simulink model "variacion_n"  (R2019b)
settings: Solver=VariableStepAuto  StartTime=0.0  StopTime=15000  RelTol=1e-3
undefined symbols (not defined in the file): n, nAum, nDis, nMitadDis, p1, p2, p3, Vi
libraries: simulink x4
settings Model: Creator=USUARIO  LastModifiedBy=USUARIO

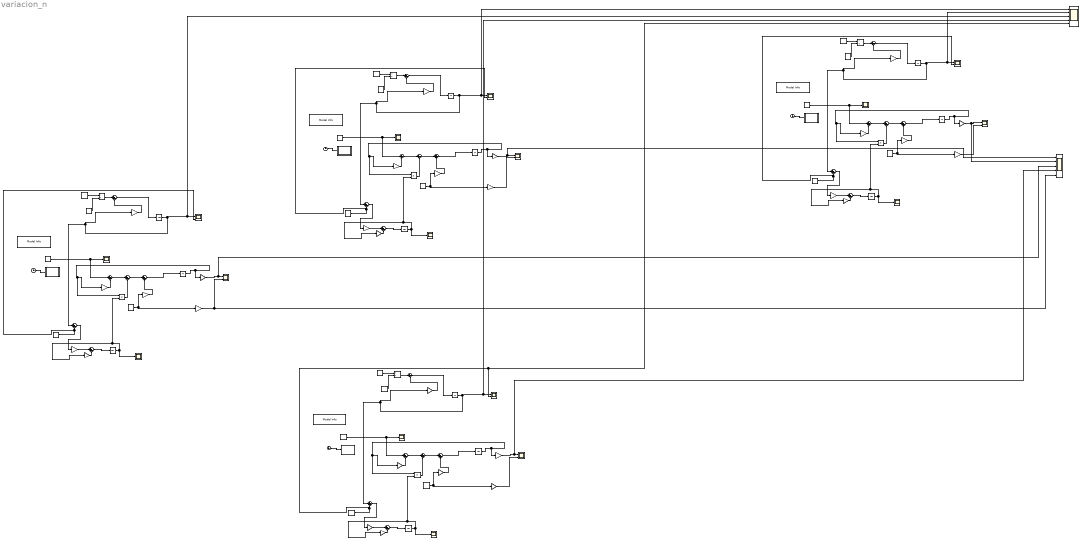
== system variacion_n ==
  Clock{1..4} (4 alike) : Clock
  Constant{1,3,5..6} (4 alike) : Constant  Value=0
  Constant{2,4,7..8} (4 alike) : Constant  Value=Vi
  Divide{1..4} (4 alike) : Product  Inputs=*/
  Gain{1,6,8,13..14,19,22,27} (8 alike) : Gain  Gain=p1
  Gain{3,5,10,12,16,18,24,26} (8 alike) : Gain  Gain=18
  Gain11 : Gain  Gain=nAum
  Gain{2,9,15,23} (4 alike) : Gain  Gain=p3
  Gain17 : Gain  Gain=n
  Gain{7,20..21,28} (4 alike) : Gain  Gain=p2
  Gain25 : Gain  Gain=nMitadDis
  Gain4 : Gain  Gain=nDis
  Glucosa basal{1..4} (4 alike) : Constant  Value=7
  Grafica ingesta D{1..4} (4 alike) : Scope
  Ingesta 75 g1 : MATLAB Function  TreatAsAtomicUnit=on
  Ingesta 75 g2 : MATLAB Function  TreatAsAtomicUnit=on
  Ingesta 75 g3 : MATLAB Function  TreatAsAtomicUnit=on
  Ingesta 75 g4 : MATLAB Function  TreatAsAtomicUnit=on
  Insulina basal{1..4} (4 alike) : Constant  Value=10
  Integrator{1,4,7,10} (4 alike) : Integrator  InitialCondition=10
  Integrator{2,5,8,11} (4 alike) : Integrator  InitialCondition=7
  Integrator{3,6,9,12} (4 alike) : Integrator  InitialCondition=-0.000194
  Model Info1 : simulink/Model-Wide Utilities/Model Info  Frame=on  DisplayStringWithTags=|  HorizontalTextAlignment=Center  LeftAlignmentValue=0.5
      | MODELO MODIFICADO
      | 
      | TRAS INGESTA CON INSULINA
      | 
      | PERSONA DIABETICA
  Model Info2 : simulink/Model-Wide Utilities/Model Info  Frame=on  DisplayStringWithTags=|  HorizontalTextAlignment=Center  LeftAlignmentValue=0.5
      | MODELO MODIFICADO
      | 
      | TRAS INGESTA CON INSULINA
      | 
      | PERSONA DIABETICA
  Model Info3 : simulink/Model-Wide Utilities/Model Info  Frame=on  DisplayStringWithTags=|  HorizontalTextAlignment=Center  LeftAlignmentValue=0.5
      | MODELO MODIFICADO
      | 
      | TRAS INGESTA CON INSULINA
      | 
      | PERSONA DIABETICA
  Model Info4 : simulink/Model-Wide Utilities/Model Info  Frame=on  DisplayStringWithTags=|  HorizontalTextAlignment=Center  LeftAlignmentValue=0.5
      | MODELO MODIFICADO
      | 
      | TRAS INGESTA CON INSULINA
      | 
      | PERSONA DIABETICA
  Product{1..4} (4 alike) : Product
  Sum{1..2,4..8,10..15,17..20,22..24} (20 alike) : Sum  Inputs=|+-
  Sum{3,9,16,21} (4 alike) : Sum  Inputs=|++
  U (ins. exógena) cte{1..4} (4 alike) : Constant  Value=0.185
  glucosa tras ingesta{1..4} (4 alike) : Scope  NumInputPorts=2
  grafica insulina{1,3..4,6} (4 alike) : Scope  NumInputPorts=2
  grafica insulina2 : Scope  NumInputPorts=5
  grafica insulina5 : Scope  NumInputPorts=5
  insulina activa{1..4} (4 alike) : Scope
  wires:
  Insulina basal4/1 -> grafica insulina1/2, Sum14/2  "insulina basal"
  Sum16/1 -> Integrator8/1
  Glucosa basal3/1 -> Gain19/1, Gain18/1  "glucosa basal"
  Product4/1 -> Sum18/2
  U (ins. exógena) cte3/1 -> Divide3/1
  Sum19/1 -> Integrator7/1
  Gain15/1 -> Sum17/1
  Gain17/1 -> Sum19/2
  Clock3/1 -> Ingesta 75 g3/1(in)
  Gain16/1 -> grafica insulina2/3, glucosa tras ingesta3/1  "Glucosa para parámetro n original"
  Divide3/1 -> Sum19/1
  Sum14/1 -> Gain15/1
  Integrator7/1 -> grafica insulina5/3, grafica insulina1/1, Gain17/1, Sum14/1  "Insulina parámetro n original"
  Sum17/1 -> Integrator9/1
  Integrator9/1 -> insulina activa3/1, Product4/2, Gain20/1  "X(t)"
  Gain18/1 -> grafica insulina2/5, glucosa tras ingesta3/2  "glucosa basal"
  Integrator8/1 -> Gain16/1, Product4/1, Gain14/1  "G(t)"
  Gain20/1 -> Sum17/2
  Constant7/1 -> Divide3/2
  Sum15/1 -> Sum18/1
  Gain19/1 -> Sum16/2
  Gain14/1 -> Sum15/2
  Constant6/1 -> Grafica ingesta D3/1, Sum15/1
  Sum18/1 -> Sum16/1
  Constant1/1 -> Grafica ingesta D1/1, Sum2/1
  Sum5/1 -> Sum3/1
  Constant2/1 -> Divide1/2
  Gain7/1 -> Sum4/2
  Gain1/1 -> Sum2/2
  Sum2/1 -> Sum5/1
  Integrator3/1 -> insulina activa1/1, Product1/2, Gain7/1  "X(t)"
  Integrator2/1 -> Gain3/1, Product1/1, Gain1/1  "G(t)"
  Sum4/1 -> Integrator3/1
  Integrator1/1 -> grafica insulina5/1, grafica insulina3/1, Gain4/1, Sum1/1  "Insulina parámetro n muy reducido"
  Gain4/1 -> Sum6/2
  Sum1/1 -> Gain2/1
  Sum6/1 -> Integrator1/1
  Gain2/1 -> Sum4/1
  Divide1/1 -> Sum6/1
  Gain5/1 -> glucosa tras ingesta1/2  "glucosa basal"
  Clock1/1 -> Ingesta 75 g1/1(in)
  Product1/1 -> Sum5/2
  Sum3/1 -> Integrator2/1
  Gain3/1 -> glucosa tras ingesta1/1, grafica insulina2/1  "Glucosa parámetro n muy reducido"
  U (ins. exógena) cte1/1 -> Divide1/1
  Glucosa basal1/1 -> Gain6/1, Gain5/1  "glucosa basal"
  Gain6/1 -> Sum3/2
  Insulina basal1/1 -> grafica insulina3/2, Sum1/2  "insulina basal"
  Constant3/1 -> Grafica ingesta D2/1, Sum8/1
  Sum11/1 -> Sum9/1
  Constant4/1 -> Divide2/2
  Gain21/1 -> Sum10/2
  Gain8/1 -> Sum8/2
  Sum8/1 -> Sum11/1
  Integrator6/1 -> insulina activa2/1, Product2/2, Gain21/1  "X(t)"
  Integrator5/1 -> Gain10/1, Product2/1, Gain8/1  "G(t)"
  Sum10/1 -> Integrator6/1
  Integrator4/1 -> grafica insulina5/4, grafica insulina4/1, Gain11/1, Sum7/1  "Insulina parámetro n aumentado"
  Gain11/1 -> Sum12/2
  Sum7/1 -> Gain9/1
  Sum12/1 -> Integrator4/1
  Gain9/1 -> Sum10/1
  Divide2/1 -> Sum12/1
  Gain12/1 -> glucosa tras ingesta2/2  "glucosa basal"
  Clock2/1 -> Ingesta 75 g2/1(in)
  Product2/1 -> Sum11/2
  Sum9/1 -> Integrator5/1
  Gain10/1 -> grafica insulina2/4, glucosa tras ingesta2/1  "Glucosa parámetro n aumentado"
  U (ins. exógena) cte2/1 -> Divide2/1
  Glucosa basal2/1 -> Gain13/1, Gain12/1  "glucosa basal"
  Gain13/1 -> Sum9/2
  Insulina basal2/1 -> grafica insulina4/2, grafica insulina5/5, Sum7/2  "insulina basal"
  Sum20/1 -> Sum23/1
  Constant5/1 -> Grafica ingesta D4/1, Sum20/1
  Insulina basal3/1 -> grafica insulina6/2, Sum13/2  "insulina basal"
  Glucosa basal4/1 -> Gain27/1, Gain26/1  "glucosa basal"
  Sum23/1 -> Sum21/1
  Gain27/1 -> Sum21/2
  Sum22/1 -> Integrator12/1
  Constant8/1 -> Divide4/2
  Integrator11/1 -> Gain24/1, Product3/1, Gain22/1  "G(t)"
  Integrator12/1 -> insulina activa4/1, Product3/2, Gain28/1  "X(t)"
  Gain22/1 -> Sum20/2
  U (ins. exógena) cte4/1 -> Divide4/1
  Gain24/1 -> grafica insulina2/2, glucosa tras ingesta4/1  "Glucosa parámetro n reducido"
  Sum21/1 -> Integrator11/1
  Clock4/1 -> Ingesta 75 g4/1(in)
  Product3/1 -> Sum23/2
  Divide4/1 -> Sum24/1
  Gain26/1 -> glucosa tras ingesta4/2  "glucosa basal"
  Gain25/1 -> Sum24/2
  Sum24/1 -> Integrator10/1
  Sum13/1 -> Gain23/1
  Gain23/1 -> Sum22/1
  Integrator10/1 -> grafica insulina5/2, grafica insulina6/1, Gain25/1, Sum13/1  "Insulina parámetro n reducido"
  Gain28/1 -> Sum22/2

== matlab function variacion_n/Ingesta 75 g1 ==
  data: in input; D output
function D = comida(in)
% Variables de entrada en la funcion
t = in(1) %- 8*60*60; % Ajuste para iniciar a las 8 de la mañana
 
% Parámetros del modelo
Ag = 0.8; % adimensional
Tmaxi = 55*60; % s
Vg = 13.79; % L
Tmaxg = 40*60; % s
t1 = 0;
Dg = 0;
f = 1000/180; % factor de conversión de g a mmol
 
% Comidas (perturbaciones) a lo largo de un día
if t >= 0 && t < 180*60 % ingesta de 75 g de HC
    t1 = 0;
    Dg = 50*f;
end
 
% Ecuación
D = (Dg*Ag*(t-t1)*exp(-(t-t1)/Tmaxi))/(Vg*Tmaxg^2);

== matlab function variacion_n/Ingesta 75 g2 ==
  data: in input; D output
function D = comida(in)
% Variables de entrada en la funcion
t = in(1) %- 8*60*60; % Ajuste para iniciar a las 8 de la mañana
 
% Parámetros del modelo
Ag = 0.8; % adimensional
Tmaxi = 55*60; % s
Vg = 13.79; % L
Tmaxg = 40*60; % s
t1 = 0;
Dg = 0;
f = 1000/180; % factor de conversión de g a mmol
 
% Comidas (perturbaciones) a lo largo de un día
if t >= 0 && t < 180*60 % ingesta de 75 g de HC
    t1 = 0;
    Dg = 50*f;
end
 
% Ecuación
D = (Dg*Ag*(t-t1)*exp(-(t-t1)/Tmaxi))/(Vg*Tmaxg^2);

== matlab function variacion_n/Ingesta 75 g3 ==
  data: in input; D output
function D = comida(in)
% Variables de entrada en la funcion
t = in(1) %- 8*60*60; % Ajuste para iniciar a las 8 de la mañana
 
% Parámetros del modelo
Ag = 0.8; % adimensional
Tmaxi = 55*60; % s
Vg = 13.79; % L
Tmaxg = 40*60; % s
t1 = 0;
Dg = 0;
f = 1000/180; % factor de conversión de g a mmol
 
% Comidas (perturbaciones) a lo largo de un día
if t >= 0 && t < 180*60 % ingesta de 75 g de HC
    t1 = 0;
    Dg = 50*f;
end
 
% Ecuación
D = (Dg*Ag*(t-t1)*exp(-(t-t1)/Tmaxi))/(Vg*Tmaxg^2);

== matlab function variacion_n/Ingesta 75 g4 ==
  data: in input; D output
function D = comida(in)
% Variables de entrada en la funcion
t = in(1) %- 8*60*60; % Ajuste para iniciar a las 8 de la mañana
 
% Parámetros del modelo
Ag = 0.8; % adimensional
Tmaxi = 55*60; % s
Vg = 13.79; % L
Tmaxg = 40*60; % s
t1 = 0;
Dg = 0;
f = 1000/180; % factor de conversión de g a mmol
 
% Comidas (perturbaciones) a lo largo de un día
if t >= 0 && t < 180*60 % ingesta de 75 g de HC
    t1 = 0;
    Dg = 50*f;
end
 
% Ecuación
D = (Dg*Ag*(t-t1)*exp(-(t-t1)/Tmaxi))/(Vg*Tmaxg^2);
